simulink model "rev0BB"  (R2017b)
settings: Solver=FixedStepDiscrete  StartTime=0  StopTime=(((preLen+100+dataLenSymbols)*1+pad_first*3)*basePer)  RelTol=1e-3
values from neighbouring files (symbols this model uses):
  ack_stf_len_symbols = length(x_ACK_STF)    [rev0BB_setup.m]
  agc_delay_lag = 32    [rev0BB_setup.m]
  agc_detector_coef = ones(1,agc_detector_taps)./agc_detector_taps    [rev0BB_setup.m]
  agc_on = true    [rev0BB_startup.m]
  agc_sat_low = -agcSaturation    (= -12)    [rev0BB_setup.m]
  agc_sat_up = agcSaturation    (= 12)    [rev0BB_setup.m]
  agcDesired = 0    [rev0BB_setup.m]
  agcExpDomain = agcSaturation    (= 12)    [rev0BB_setup.m]
  agcExpResolution = 2^-5    (= 0.03125)    [rev0BB_setup.m]
  agcPwrAvgNum = 128    [rev0BB_setup.m]
  agcSaturation = 12    [rev0BB_setup.m]
  agcSettleThresh = 0.65    [rev0BB_setup.m]
  agcStep = 2^-8    (= 0.00390625)    [rev0BB_setup.m]
  atanDomain = 5    [rev0BB_setup.m]
  atanDomainTiming = 256    [rev0BB_setup.m]
  atanResolution = 2^-9    (= 0.001953125)    [rev0BB_setup.m]
  atanResolutionTiming = 2^-5    (= 0.03125)    [rev0BB_setup.m]
  averaging_num = ones(1, averaging_samples)    [rev0BB_setup.m]
  averaging_samples = 128    [rev0BB_setup.m]
  awgnSeed = abs(dBSnrRange(dBSnrInd)*1000+trial+10000000)    [plotBer.m]    (also in rev0BB_startup.m = 67)
  basePer = 1/baseFreq    (= 5e-08)    [rev0BB_setup.m]
  bitsPerSymbolHeader = log2(radixHeader)    [rev0BB_setup.m]
  bitsPerSymbolMax = log2(radixMax)    [rev0BB_setup.m]
  cal_sig_i_mult = 1.0    (= 1)    [rev0BB_startup.m]
  cal_sig_i_offset = 0.0    (= 0)    [rev0BB_startup.m]
  cal_sig_q_mult = 1.0    (= 1)    [rev0BB_startup.m]
  cal_sig_q_offset = 0.0    (= 0)    [rev0BB_startup.m]
  cefEarlyWarning = 256    [rev0BB_setup.m]
  cefLen = length(x_CEF)    [rev0BB_setup.m]
  channelFIR = zeros(1, round(maxSampleDelay)+1)    [rev0BB_startup.m]
  coarseCFOAdaptDelay = 1    [rev0BB_setup.m]
  cr_i = 0.020    (= 0.02)    [rev0BB_setup.m]
  cr_i_preamp = 2^-9    (= 0.001953125)    [rev0BB_setup.m]
  cr_int1_sat_low = -cr_integrator1_saturation    (= -0.6)    [rev0BB_setup.m]
  cr_int1_sat_up = cr_integrator1_saturation    (= 0.6)    [rev0BB_setup.m]
  cr_integrator1_decay = 1    [rev0BB_setup.m]
  cr_integrator1_saturation = 0.6    [rev0BB_setup.m]
  cr_mult_pipeline = 0    [rev0BB_setup.m]
  cr_p = 0.015    [rev0BB_setup.m]
  cr_sat2_low = -cr_saturation2    (= -0.6)    [rev0BB_setup.m]
  cr_sat2_up = cr_saturation2    (= 0.6)    [rev0BB_setup.m]
  cr_smooth_num = (1/cr_smooth_samples).*ones(1, cr_smooth_samples)    [rev0BB_setup.m]
  D_128 = [ 1,  8,  2,  4, 16, 32, 64]    [golay.m]    (also in rev0BB_setup.m)
  D_32 = [ 1,  4,  8,  2, 16]    [golay.m]    (also in rev0BB_setup.m)
  dataLenSymbols = header_len_bytes*8/bitsPerSymbolHeader + frame_len_bytes*8/bitsPerSymbol    [rev0BB_setup.m]
  default_channel = 3    [rev0BB_setup.m]
  dmm_coefs = ones(1,dmm_samples)./dmm_samples    [rev0BB_setup.m]
  dst_field_len = 8    [rev0BB_setup.m]
  expDomain = 3.3    [rev0BB_setup.m]
  expResolution = 2^-5    (= 0.03125)    [rev0BB_setup.m]
  expTol = .1    (= 0.1)    [rev0BB_setup.m]
  flush_delay = regular_pipeline*2+mult_pipeline+4    (= 4)    [rev0BB_setup.m]
  frac_lut_domain = 256    [rev0BB_setup.m]
  frac_lut_domain_cr = 64    [rev0BB_setup.m]
  frac_lut_range_max = 512    [rev0BB_setup.m]
  frac_lut_range_max_coarse_cfo = 127    [rev0BB_setup.m]
  frac_lut_range_max_cr = 127    [rev0BB_setup.m]
  frac_lut_range_min = -frac_lut_range_max    (= -512)    [rev0BB_setup.m]
  frac_lut_range_min_coarse_cfo = -frac_lut_range_max_coarse_cfo    (= -127)    [rev0BB_setup.m]
  frac_lut_range_min_cr = -frac_lut_range_max_cr    (= -127)    [rev0BB_setup.m]
  frac_lut_table_breaks = -frac_lut_domain:frac_lut_res:(frac_lut_domain-1)    [rev0BB_setup.m]
  frac_lut_table_breaks_coarse_cfo = -frac_lut_domain_coarse_cfo:frac_lut_res_coarse_cfo:(frac_lut_domain_coarse_cfo-1)    [rev0BB_setup.m]
  frac_lut_table_breaks_cr = -frac_lut_domain_cr:frac_lut_res_cr:(frac_lut_domain_cr-1)    [rev0BB_setup.m]
  frac_lut_table_data = 1./frac_lut_table_breaks    [rev0BB_setup.m]
  frac_lut_table_data_coarse_cfo = 1./frac_lut_table_breaks_coarse_cfo    [rev0BB_setup.m]
  frac_lut_table_data_cr = 1./frac_lut_table_breaks_cr    [rev0BB_setup.m]
  freeze_en_agc = true    [rev0BB_startup.m]
  freeze_en_cr_int1 = false    [rev0BB_startup.m]
  freeze_en_cr_int2 = false    [rev0BB_startup.m]
  freeze_en_cr_phase = false    [rev0BB_startup.m]
  freeze_en_tr_int1 = false    [rev0BB_startup.m]
  freeze_en_tr_int2 = false    [rev0BB_startup.m]
  freeze_en_tr_phase = false    [rev0BB_startup.m]
  freeze_on_cef_done = true    [rev0BB_startup.m]
  freeze_on_stf_done = false    [rev0BB_startup.m]
  freeze_on_valid = true    [rev0BB_startup.m]
  golay_type = 32    [rev0BB_setup.m]
  guardInt = int16(4)    [rev0BB_setup.m]
  guardTol = int16(5)    [rev0BB_setup.m]
  header_len_bytes = 8    [rev0BB_setup.m]
  lineWidth = 60    [rev0BB_setup.m]
  lmsEqDepth = 38    [rev0BB_setup.m]
  lmsStep_init = 0.006    [rev0BB_setup.m]
  lmsStep_meta = (lmsStep_final - lmsStep_init)/cefLen    [rev0BB_setup.m]
  lnDomain = 16    [rev0BB_setup.m]
  lnResolution = 2^-5    (= 0.03125)    [rev0BB_setup.m]
  local_node_id = 2    [rev0BB_startup.m]
  maxMsgSize = length(xSpectrum_PRE)+dataLenSymbols+300    [rev0BB_setup.m]
  minSTFPeaks = 3    [rev0BB_setup.m]
  mod_scheme_len_bytes = 1    [rev0BB_setup.m]
  modBPS = [1, 2, 4]    [rev0BB_setup.m]
  modKeys = [0, 1, 2]    [rev0BB_setup.m]
  mult_pipeline = 0    [rev0BB_setup.m]
  overSampleFreq = 80e6    (= 80000000)    [rev0BB_setup.m]
  overSamplePer = 1/overSampleFreq    (= 1.25e-08)    [rev0BB_setup.m]
  pad_first = 1000    [createTestVectors.m]
  post_cr_i_offset = 0    [rev0BB_startup.m]
  post_cr_q_offset = 0    [rev0BB_startup.m]
  preambleSequentialDetect = 2    [rev0BB_setup.m]
  preLen = length(x_PRE)    [rev0BB_setup.m]
  qam16_demod_scale_factor = qam16_hdl_distance/qam16_power_normalized_distance    [rev0BB_setup.m]
  rcRxFilt = [0.000303163120401141 -0.00118915940834234 -0.00187387637177 -0.00124167532697737 0.00029186889076529 0.00164526160586517 0.00182432050803312 0.000652133621739543 -0.00105668254004908 -0.00204011570659167 -0.00150058088768918 0.00026138356356816 0.0019831869994874 0.00231075800085521 0.000821993419120097 -0.00154687337975486 -0.00305430783933469 -0.00238186490079127 0.000301216962040692 0.00325307 ...(+2001 chars)    [rev0BB_setup.m]
  rcTxFilt = [0.000303163120401141 -0.00118915940834234 -0.00187387637177 -0.00124167532697737 0.00029186889076529 0.00164526160586517 0.00182432050803312 0.000652133621739543 -0.00105668254004908 -0.00204011570659167 -0.00150058088768918 0.00026138356356816 0.0019831869994874 0.00231075800085521 0.000821993419120097 -0.00154687337975486 -0.00305430783933469 -0.00238186490079127 0.000301216962040692 0.00325307 ...(+2001 chars)    [rev0BB_setup.m]
  regular_pipeline = 0    [rev0BB_setup.m]
  rx_gain = 1    [rev0BB_setup.m]
  rx_gain_i = 1    [rev0BB_setup.m]
  rx_gain_q = 1    [rev0BB_setup.m]
  rx_impare_i_offset = 0    [rev0BB_startup.m]
  rx_impare_i_scale = 1    [rev0BB_startup.m]
  rx_impare_q_offset = 0    [rev0BB_startup.m]
  rx_impare_q_scale = 1    [rev0BB_startup.m]
  rx_offset_correction_i = 0    [rev0BB_startup.m]
  rx_offset_correction_q = 0    [rev0BB_startup.m]
  sin_source_amp = 1    [rev0BB_setup.m]
  sin_source_freq = 250e6/16    (= 15625000)    [rev0BB_setup.m]
  slowPer = overSamplePer*slowSample    (= 2.5e-08)    [rev0BB_setup.m]
  std_pkt_type = 0    [rev0BB_setup.m]
  stfLen = length(x_STF)    [rev0BB_setup.m]
  testMsg = cat(1, xCTRL_PRE_adj, header, payload)    [plotBer.m]
  timing_i = 0.25    [rev0BB_setup.m]
  ... (+25 more)
undefined symbols (not defined in the file or in its folder): cr_integrator2_saturation, doppler, i, magnitude, useFadingChannel
libraries: helperLib x128, simulink x90, golayLib x34, dspsigops x32, commfilt2 x27, commdigbbndpm3 x8, hdlsllib x6, dsparch4 x4, commdigbbndam3 x4, commchan3 x2, commrflib2 x2, commcrc2 x2
(part 4 of 10)

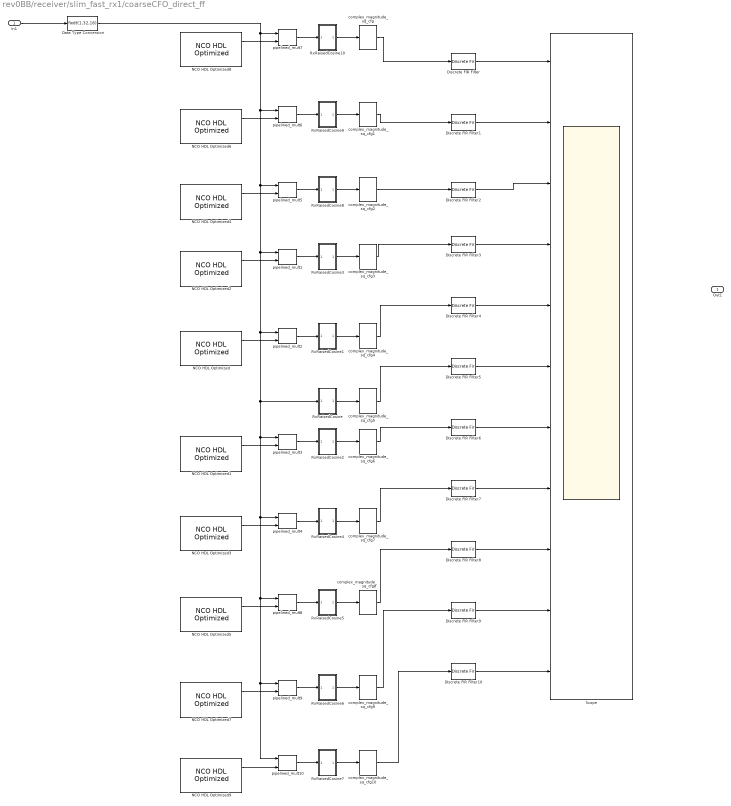
== system rev0BB/receiver/slim_fast_rx1/coarseCFO_direct_ff ==
  In1 : Inport
  Data Type Conversion : DataTypeConversion  OutDataTypeStr=fixdt(1,32,16)
  Discrete FIR Filter{,1..10} (11 alike) : DiscreteFir  Coefficients=ones(1,512)./512
  NCO HDL Optimized : dspsigops/NCO HDL Optimized  PhaseIncrementSource=Property  PhaseIncrement=floor(1000*2^17/overSampleFreq)  PhaseOffsetSource=Property  PhaseOffset=0  DitherSource=Property  NumDitherBits=4  PhaseQuantization=on  NumQuantizerAccumulatorBits=17  LUTCompress=on  ResetAction=off  ValidInputPort=off  Waveform=Complex exponential  PhasePort=off  SimulateUsing=Code generation  AccumulatorWL=21  OutputDataType=Binary point scaling  OutputWL=18  OutputFL=11
      settings: SourceProductName=DSP System Toolbox  SourceProductBaseCode=DS
  NCO HDL Optimized1 : dspsigops/NCO HDL Optimized  PhaseIncrementSource=Property  PhaseIncrement=-floor(1000*2^17/overSampleFreq)  PhaseOffsetSource=Property  PhaseOffset=0  DitherSource=Property  NumDitherBits=4  PhaseQuantization=on  NumQuantizerAccumulatorBits=17  LUTCompress=on  ResetAction=off  ValidInputPort=off  Waveform=Complex exponential  PhasePort=off  SimulateUsing=Code generation  AccumulatorWL=21  OutputDataType=Binary point scaling  OutputWL=18  OutputFL=11
      settings: SourceProductName=DSP System Toolbox  SourceProductBaseCode=DS
  NCO HDL Optimized2 : dspsigops/NCO HDL Optimized  PhaseIncrementSource=Property  PhaseIncrement=floor(2000*2^17/overSampleFreq)  PhaseOffsetSource=Property  PhaseOffset=0  DitherSource=Property  NumDitherBits=4  PhaseQuantization=on  NumQuantizerAccumulatorBits=17  LUTCompress=on  ResetAction=off  ValidInputPort=off  Waveform=Complex exponential  PhasePort=off  SimulateUsing=Code generation  AccumulatorWL=21  OutputDataType=Binary point scaling  OutputWL=18  OutputFL=11
      settings: SourceProductName=DSP System Toolbox  SourceProductBaseCode=DS
  NCO HDL Optimized3 : dspsigops/NCO HDL Optimized  PhaseIncrementSource=Property  PhaseIncrement=-floor(2000*2^17/overSampleFreq)  PhaseOffsetSource=Property  PhaseOffset=0  DitherSource=Property  NumDitherBits=4  PhaseQuantization=on  NumQuantizerAccumulatorBits=17  LUTCompress=on  ResetAction=off  ValidInputPort=off  Waveform=Complex exponential  PhasePort=off  SimulateUsing=Code generation  AccumulatorWL=21  OutputDataType=Binary point scaling  OutputWL=18  OutputFL=11
      settings: SourceProductName=DSP System Toolbox  SourceProductBaseCode=DS
  NCO HDL Optimized4 : dspsigops/NCO HDL Optimized  PhaseIncrementSource=Property  PhaseIncrement=floor(3000*2^17/overSampleFreq)  PhaseOffsetSource=Property  PhaseOffset=0  DitherSource=Property  NumDitherBits=4  PhaseQuantization=on  NumQuantizerAccumulatorBits=17  LUTCompress=on  ResetAction=off  ValidInputPort=off  Waveform=Complex exponential  PhasePort=off  SimulateUsing=Code generation  AccumulatorWL=21  OutputDataType=Binary point scaling  OutputWL=18  OutputFL=11
      settings: SourceProductName=DSP System Toolbox  SourceProductBaseCode=DS
  NCO HDL Optimized5 : dspsigops/NCO HDL Optimized  PhaseIncrementSource=Property  PhaseIncrement=floor(-3000*2^17/overSampleFreq)  PhaseOffsetSource=Property  PhaseOffset=0  DitherSource=Property  NumDitherBits=4  PhaseQuantization=on  NumQuantizerAccumulatorBits=17  LUTCompress=on  ResetAction=off  ValidInputPort=off  Waveform=Complex exponential  PhasePort=off  SimulateUsing=Code generation  AccumulatorWL=21  OutputDataType=Binary point scaling  OutputWL=18  OutputFL=11
      settings: SourceProductName=DSP System Toolbox  SourceProductBaseCode=DS
  NCO HDL Optimized6 : dspsigops/NCO HDL Optimized  PhaseIncrementSource=Property  PhaseIncrement=floor(4000*2^17/overSampleFreq)  PhaseOffsetSource=Property  PhaseOffset=0  DitherSource=Property  NumDitherBits=4  PhaseQuantization=on  NumQuantizerAccumulatorBits=17  LUTCompress=on  ResetAction=off  ValidInputPort=off  Waveform=Complex exponential  PhasePort=off  SimulateUsing=Code generation  AccumulatorWL=21  OutputDataType=Binary point scaling  OutputWL=18  OutputFL=11
      settings: SourceProductName=DSP System Toolbox  SourceProductBaseCode=DS
  NCO HDL Optimized7 : dspsigops/NCO HDL Optimized  PhaseIncrementSource=Property  PhaseIncrement=-floor(4000*2^17/overSampleFreq)  PhaseOffsetSource=Property  PhaseOffset=0  DitherSource=Property  NumDitherBits=4  PhaseQuantization=on  NumQuantizerAccumulatorBits=17  LUTCompress=on  ResetAction=off  ValidInputPort=off  Waveform=Complex exponential  PhasePort=off  SimulateUsing=Code generation  AccumulatorWL=21  OutputDataType=Binary point scaling  OutputWL=18  OutputFL=11
      settings: SourceProductName=DSP System Toolbox  SourceProductBaseCode=DS
  NCO HDL Optimized8 : dspsigops/NCO HDL Optimized  PhaseIncrementSource=Property  PhaseIncrement=floor(5000*2^17/overSampleFreq)  PhaseOffsetSource=Property  PhaseOffset=0  DitherSource=Property  NumDitherBits=4  PhaseQuantization=on  NumQuantizerAccumulatorBits=17  LUTCompress=on  ResetAction=off  ValidInputPort=off  Waveform=Complex exponential  PhasePort=off  SimulateUsing=Code generation  AccumulatorWL=21  OutputDataType=Binary point scaling  OutputWL=18  OutputFL=11
      settings: SourceProductName=DSP System Toolbox  SourceProductBaseCode=DS
  NCO HDL Optimized9 : dspsigops/NCO HDL Optimized  PhaseIncrementSource=Property  PhaseIncrement=-floor(5000*2^17/overSampleFreq)  PhaseOffsetSource=Property  PhaseOffset=0  DitherSource=Property  NumDitherBits=4  PhaseQuantization=on  NumQuantizerAccumulatorBits=17  LUTCompress=on  ResetAction=off  ValidInputPort=off  Waveform=Complex exponential  PhasePort=off  SimulateUsing=Code generation  AccumulatorWL=21  OutputDataType=Binary point scaling  OutputWL=18  OutputFL=11
      settings: SourceProductName=DSP System Toolbox  SourceProductBaseCode=DS
  RxRaisedCosine : Subsystem
  RxRaisedCosine1 : Subsystem
  RxRaisedCosine10 : Subsystem
  RxRaisedCosine2 : Subsystem
  RxRaisedCosine3 : Subsystem
  RxRaisedCosine4 : Subsystem
  RxRaisedCosine5 : Subsystem
  RxRaisedCosine6 : Subsystem
  RxRaisedCosine7 : Subsystem
  RxRaisedCosine8 : Subsystem
  RxRaisedCosine9 : Subsystem
  Scope : Scope  NumInputPorts=11
  complex_magnitude_sq_cfg{,1..10} (11 alike) : helperLib/complex_magnitude_sq_cfg  mult=mult_pipeline  pipe=regular_pipeline
  pipelined_mult{1..10} (10 alike) : helperLib/pipelined_mult  d=wide_mult_pipeline
  Out1 : Outport
  wires:
  NCO HDL Optimized/1 -> pipelined_mult2/2
  NCO HDL Optimized1/1 -> pipelined_mult3/2
  pipelined_mult3/1 -> RxRaisedCosine2/1(In2)
  pipelined_mult2/1 -> RxRaisedCosine1/1(In2)
  NCO HDL Optimized6/1 -> pipelined_mult6/2
  NCO HDL Optimized4/1 -> pipelined_mult5/2
  NCO HDL Optimized2/1 -> pipelined_mult1/2
  pipelined_mult1/1 -> RxRaisedCosine3/1(In2)
  NCO HDL Optimized8/1 -> pipelined_mult7/2
  In1/1 -> Data Type Conversion/1
  NCO HDL Optimized3/1 -> pipelined_mult4/2
  NCO HDL Optimized5/1 -> pipelined_mult8/2
  NCO HDL Optimized7/1 -> pipelined_mult9/2
  NCO HDL Optimized9/1 -> pipelined_mult10/2
  pipelined_mult4/1 -> RxRaisedCosine4/1(In2)
  pipelined_mult8/1 -> RxRaisedCosine5/1(In2)
  pipelined_mult9/1 -> RxRaisedCosine6/1(In2)
  pipelined_mult10/1 -> RxRaisedCosine7/1(In2)
  pipelined_mult5/1 -> RxRaisedCosine8/1(In2)
  pipelined_mult6/1 -> RxRaisedCosine9/1(In2)
  pipelined_mult7/1 -> RxRaisedCosine10/1(In2)
  RxRaisedCosine10/1(Out2) -> complex_magnitude_sq_cfg/1
  RxRaisedCosine9/1(Out2) -> complex_magnitude_sq_cfg1/1
  RxRaisedCosine8/1(Out2) -> complex_magnitude_sq_cfg2/1
  RxRaisedCosine3/1(Out2) -> complex_magnitude_sq_cfg3/1
  RxRaisedCosine1/1(Out2) -> complex_magnitude_sq_cfg4/1
  RxRaisedCosine/1(Out2) -> complex_magnitude_sq_cfg5/1
  RxRaisedCosine2/1(Out2) -> complex_magnitude_sq_cfg6/1
  RxRaisedCosine4/1(Out2) -> complex_magnitude_sq_cfg7/1
  RxRaisedCosine5/1(Out2) -> complex_magnitude_sq_cfg8/1
  RxRaisedCosine6/1(Out2) -> complex_magnitude_sq_cfg9/1
  RxRaisedCosine7/1(Out2) -> complex_magnitude_sq_cfg10/1
  complex_magnitude_sq_cfg/1 -> Discrete FIR Filter/1
  complex_magnitude_sq_cfg1/1 -> Discrete FIR Filter1/1
  complex_magnitude_sq_cfg2/1 -> Discrete FIR Filter2/1
  complex_magnitude_sq_cfg3/1 -> Discrete FIR Filter3/1
  complex_magnitude_sq_cfg4/1 -> Discrete FIR Filter4/1
  complex_magnitude_sq_cfg5/1 -> Discrete FIR Filter5/1
  complex_magnitude_sq_cfg6/1 -> Discrete FIR Filter6/1
  complex_magnitude_sq_cfg7/1 -> Discrete FIR Filter7/1
  complex_magnitude_sq_cfg8/1 -> Discrete FIR Filter8/1
  complex_magnitude_sq_cfg9/1 -> Discrete FIR Filter9/1
  complex_magnitude_sq_cfg10/1 -> Discrete FIR Filter10/1
  Data Type Conversion/1 -> pipelined_mult7/1, pipelined_mult6/1, pipelined_mult5/1, pipelined_mult1/1, RxRaisedCosine/1(In2), pipelined_mult10/1, pipelined_mult9/1, pipelined_mult8/1, pipelined_mult4/1, pipelined_mult3/1, pipelined_mult2/1
  Discrete FIR Filter/1 -> Scope/1
  Discrete FIR Filter1/1 -> Scope/2
  Discrete FIR Filter2/1 -> Scope/3
  Discrete FIR Filter3/1 -> Scope/4
  Discrete FIR Filter4/1 -> Scope/5
  Discrete FIR Filter5/1 -> Scope/6
  Discrete FIR Filter6/1 -> Scope/7
  Discrete FIR Filter7/1 -> Scope/8
  Discrete FIR Filter8/1 -> Scope/9
  Discrete FIR Filter9/1 -> Scope/10
  Discrete FIR Filter10/1 -> Scope/11

== system rev0BB/receiver/slim_fast_rx1/coarseCFO_ff ==
  note: The frequency estemator is derived in Ch 8.2.2 (Pg 457-462) in
      | Digital Communication Recievers: Syncronization, Channel Estimation, and Signal Processing by Meyr et al.
  SignalIn : Inport
  Coarse_CFO_EST : Scope
  Complex to Real-Imag : ComplexToRealImag
  Constant : Constant  Value=0  OutDataTypeStr=int16
  Constant1 : Constant  Value=true  OutDataTypeStr=boolean
  Data Type Conversion : DataTypeConversion  OutDataTypeStr=double
  Data Type Conversion1 : DataTypeConversion  OutDataTypeStr=double
  Delay : Delay  DelayLength=1  InitialCondition=0
  Discrete FIR Filter : DiscreteFir  Coefficients=ones(1, 4096)  AccumDataTypeStr=Inherit: Same as product output
  Gain : Gain  Gain=overSampleFreq/(2*pi)
  NCO HDL Optimized : dspsigops/NCO HDL Optimized  PhaseIncrementSource=Input port  PhaseIncrement=100  PhaseOffsetSource=Property  PhaseOffset=0  DitherSource=Property  NumDitherBits=4  PhaseQuantization=on  NumQuantizerAccumulatorBits=12  LUTCompress=on  ResetAction=off  ValidInputPort=on  Waveform=Complex exponential  PhasePort=off  SimulateUsing=Code generation  AccumulatorWL=14  OutputDataType=Binary point scaling  OutputWL=14  OutputFL=11
      settings: SourceProductName=DSP System Toolbox  SourceProductBaseCode=DS
  Product : Product
  Trigonometric Function : Trigonometry  Operator=atan2
  complex_conj : helperLib/complex_conj
  pipeline_delay : Delay  DelayLength=regular_pipeline
  pipelined_mult1 : helperLib/pipelined_mult  d=wide_mult_pipeline
  SignalOut : Outport
  wires:
  NCO HDL Optimized/1 -> pipelined_mult1/2
  SignalIn/1 -> pipeline_delay/1, pipelined_mult1/1
  pipelined_mult1/1 -> SignalOut/1
  Constant1/1 -> NCO HDL Optimized/2
  Delay/1 -> complex_conj/1
  pipeline_delay/1 -> Data Type Conversion/1, Delay/1
  Constant/1 -> NCO HDL Optimized/1
  Trigonometric Function/1 -> Gain/1
  complex_conj/1 -> Data Type Conversion1/1
  Data Type Conversion1/1 -> Product/1
  Data Type Conversion/1 -> Product/2
  Product/1 -> Discrete FIR Filter/1
  Discrete FIR Filter/1 -> Complex to Real-Imag/1
  Complex to Real-Imag/2 -> Trigonometric Function/1
  Complex to Real-Imag/1 -> Trigonometric Function/2
  Gain/1 -> Coarse_CFO_EST/1

== system rev0BB/receiver/slim_fast_rx2/AGC ==
  note: Intentionally let width grow due to distinct chance of overflow
  In : Inport
  Desired : Inport  Port=2
  Step : Inport  Port=3
  freeze : Inport  Port=4  OutDataTypeStr=boolean
  agc_sat_up : Inport  Port=5
  agc_sat_low : Inport  Port=6
  Bit Shift : hdlsllib/Logic and Bit Operations/Bit Shift  Commented=on  mode=Shift Left Logical  N=1
      settings: SourceProductName=HDL Coder  SourceProductBaseCode=HD
  Constant : Constant  Value=0  OutDataTypeStr=Inherit: Inherit via back propagation  SampleTime=-1
  Data Type Duplicate : DataTypeDuplicate  Commented=on
  Data Type Duplicate1 : DataTypeDuplicate
  Data Type Conversion1 : DataTypeConversion  OutDataTypeStr=fixdt(1,38,18)
  Delay : Delay  DelayLength=1  InitialCondition=0
  Delay1 : Delay  DelayLength=1  InitialCondition=0
  Discrete FIR Filter : DiscreteFir  FilterStructure=Direct form transposed  Coefficients=agc_detector_coef  InputProcessing=Columns as channels (frame based)  OutDataTypeStr=Inherit: Same as input
  Product : Product  Commented=on
  Saturation : Saturate  Commented=on  UpperLimit=agcSaturation  LowerLimit=-agcSaturation
  Saturation Dynamic : simulink/Discontinuities/Saturation Dynamic  OutMin=[]  OutMax=[]  OutDataTypeStr=Inherit: Same as second input  OutDataType=fixdt(1, 16)  OutScaling=2^-10  DoSatur=off
  Sum : Sum  Inputs=-+
  Sum1 : Sum  Inputs=|++
  Switch : Switch  Criteria=u2 > Threshold
  Switch1 : Switch  Criteria=u2 > Threshold
  complex_magnitude_sq_cfg : helperLib/complex_magnitude_sq_cfg  mult=wide_mult_pipeline  pipe=regular_pipeline
  exp : Subsystem
  exp1 : Subsystem  Commented=on
  ln1 : Subsystem
  mult_delay1 : Delay  Commented=on  DelayLength=wide_mult_pipeline
  pipeline_delay{,1..2,4,7..13} (11 alike) : Delay  DelayLength=regular_pipeline
  pipeline_delay3 : Delay  Commented=on  DelayLength=regular_pipeline
  pipeline_delay5 : Delay  Commented=on  DelayLength=regular_pipeline
  pipeline_delay6 : Delay  DelayLength=regular_pipeline*2
  pipelined_mult2 : helperLib/pipelined_mult  d=wide_mult_pipeline
  Correction : Outport
  LnPwr : Outport  Port=2
  wires:
  In/1 -> Data Type Conversion1/1
  Data Type Conversion1/1 -> pipeline_delay6/1
  complex_magnitude_sq_cfg/1 -> pipeline_delay9/1
  ln1/1(Out) -> pipeline_delay10/1
  Sum/1 -> pipeline_delay/1
  pipeline_delay/1 -> pipelined_mult2/2
  pipeline_delay7/1 -> pipelined_mult2/1
  Bit Shift/1 -> pipeline_delay3/1
  Sum1/1 -> Delay/1
  exp1/1(Out) -> pipeline_delay5/1
  pipeline_delay5/1 -> Data Type Duplicate/2, Product/2
  exp/1(Out) -> pipeline_delay4/1
  pipeline_delay4/1 -> Data Type Duplicate1/1, Correction/1
  Step/1 -> pipeline_delay7/1
  Desired/1 -> pipeline_delay8/1
  pipeline_delay10/1 -> LnPwr/1, Sum/1
  pipeline_delay2/1 -> exp/1(In)
  pipeline_delay3/1 -> exp1/1(In)
  pipeline_delay8/1 -> Sum/2
  pipeline_delay1/1 -> Data Type Duplicate1/2, ln1/2(data_type), Data Type Duplicate/1, Product/1, ln1/1(In)
  Saturation Dynamic/1 -> Sum1/2, Switch/3
  pipelined_mult2/1 -> Switch1/3
  Product/1 -> mult_delay1/1
  Switch/1 -> Bit Shift/1, pipeline_delay2/1, Delay1/1
  freeze/1 -> pipeline_delay13/1
  Delay1/1 -> Switch/1
  agc_sat_up/1 -> pipeline_delay11/1
  agc_sat_low/1 -> pipeline_delay12/1
  Delay/1 -> Saturation Dynamic/2
  pipeline_delay9/1 -> Discrete FIR Filter/1
  Discrete FIR Filter/1 -> pipeline_delay1/1
  pipeline_delay6/1 -> complex_magnitude_sq_cfg/1
  pipeline_delay11/1 -> Saturation Dynamic/1
  pipeline_delay12/1 -> Saturation Dynamic/3
  pipeline_delay13/1 -> Switch1/2, Switch/2
  Switch1/1 -> Sum1/1
  Constant/1 -> Switch1/1

== system rev0BB/receiver/slim_fast_rx2/Golay Correlator 128 ==
  In : Inport
  GolayCoralatorBase_fp : golayLib/GolayCoralatorBase_fp  dSub=D_128(1)*4  wSub=W_128(1)  mult=0
  GolayCoralatorBase_fp1 : golayLib/GolayCoralatorBase_fp  dSub=D_128(2)*4  wSub=W_128(2)  mult=0
  GolayCoralatorBase_fp2 : golayLib/GolayCoralatorBase_fp  dSub=D_128(3)*4  wSub=W_128(3)  mult=0
  GolayCoralatorBase_fp3 : golayLib/GolayCoralatorBase_fp  dSub=D_128(4)*4  wSub=W_128(4)  mult=0
  GolayCoralatorBase_fp4 : golayLib/GolayCoralatorBase_fp  dSub=D_128(5)*4  wSub=W_128(5)  mult=0
  GolayCoralatorBase_fp5 : golayLib/GolayCoralatorBase_fp  dSub=D_128(6)*4  wSub=W_128(6)  mult=0
  GolayCoralatorBase_fp6 : golayLib/GolayCoralatorBase_fp  dSub=D_128(7)*4  wSub=W_128(7)  mult=0
  pipeline_delay{,1..13} (14 alike) : Delay  DelayLength=regular_pipeline
  Ca : Outport
  Cb : Outport  Port=2
  wires:
  GolayCoralatorBase_fp/1 -> pipeline_delay/1
  GolayCoralatorBase_fp/2 -> pipeline_delay1/1
  GolayCoralatorBase_fp1/1 -> pipeline_delay2/1
  GolayCoralatorBase_fp1/2 -> pipeline_delay3/1
  GolayCoralatorBase_fp4/1 -> pipeline_delay8/1
  GolayCoralatorBase_fp2/1 -> pipeline_delay4/1
  GolayCoralatorBase_fp2/2 -> pipeline_delay5/1
  GolayCoralatorBase_fp3/1 -> pipeline_delay6/1
  GolayCoralatorBase_fp3/2 -> pipeline_delay7/1
  GolayCoralatorBase_fp5/2 -> pipeline_delay11/1
  GolayCoralatorBase_fp5/1 -> pipeline_delay10/1
  GolayCoralatorBase_fp6/1 -> pipeline_delay12/1
  In/1 -> GolayCoralatorBase_fp/2, GolayCoralatorBase_fp/1
  pipeline_delay/1 -> GolayCoralatorBase_fp1/1
  pipeline_delay1/1 -> GolayCoralatorBase_fp1/2
  pipeline_delay2/1 -> GolayCoralatorBase_fp2/1
  pipeline_delay3/1 -> GolayCoralatorBase_fp2/2
  pipeline_delay4/1 -> GolayCoralatorBase_fp3/1
  pipeline_delay6/1 -> GolayCoralatorBase_fp4/1
  pipeline_delay8/1 -> GolayCoralatorBase_fp5/1
  pipeline_delay10/1 -> GolayCoralatorBase_fp6/1
  pipeline_delay12/1 -> Ca/1
  pipeline_delay13/1 -> Cb/1
  pipeline_delay5/1 -> GolayCoralatorBase_fp3/2
  pipeline_delay7/1 -> GolayCoralatorBase_fp4/2
  GolayCoralatorBase_fp4/2 -> pipeline_delay9/1
  pipeline_delay9/1 -> GolayCoralatorBase_fp5/2
  pipeline_delay11/1 -> GolayCoralatorBase_fp6/2
  GolayCoralatorBase_fp6/2 -> pipeline_delay13/1

== system rev0BB/receiver/slim_fast_rx2/Golay Correlator 32 ==
  In : Inport
  GolayCoralatorBase_fp : golayLib/GolayCoralatorBase_fp  dSub=D_32(1)*4  wSub=W_32(1)  mult=0
  GolayCoralatorBase_fp1 : golayLib/GolayCoralatorBase_fp  dSub=D_32(2)*4  wSub=W_32(2)  mult=0
  GolayCoralatorBase_fp2 : golayLib/GolayCoralatorBase_fp  dSub=D_32(3)*4  wSub=W_32(3)  mult=0
  GolayCoralatorBase_fp3 : golayLib/GolayCoralatorBase_fp  dSub=D_32(4)*4  wSub=W_32(4)  mult=0
  GolayCoralatorBase_fp4 : golayLib/GolayCoralatorBase_fp  dSub=D_32(5)*4  wSub=W_32(5)  mult=0
  pipeline_delay{,1..13} (14 alike) : Delay  DelayLength=regular_pipeline
  Ca : Outport
  Cb : Outport  Port=2
  wires:
  GolayCoralatorBase_fp/1 -> pipeline_delay/1
  GolayCoralatorBase_fp/2 -> pipeline_delay1/1
  GolayCoralatorBase_fp1/1 -> pipeline_delay2/1
  GolayCoralatorBase_fp1/2 -> pipeline_delay3/1
  GolayCoralatorBase_fp4/1 -> pipeline_delay8/1
  GolayCoralatorBase_fp2/1 -> pipeline_delay4/1
  GolayCoralatorBase_fp2/2 -> pipeline_delay5/1
  GolayCoralatorBase_fp3/1 -> pipeline_delay6/1
  GolayCoralatorBase_fp3/2 -> pipeline_delay7/1
  pipeline_delay9/1 -> pipeline_delay11/1
  pipeline_delay8/1 -> pipeline_delay10/1
  pipeline_delay10/1 -> pipeline_delay12/1
  In/1 -> GolayCoralatorBase_fp/2, GolayCoralatorBase_fp/1
  pipeline_delay/1 -> GolayCoralatorBase_fp1/1
  pipeline_delay1/1 -> GolayCoralatorBase_fp1/2
  pipeline_delay2/1 -> GolayCoralatorBase_fp2/1
  pipeline_delay3/1 -> GolayCoralatorBase_fp2/2
  pipeline_delay4/1 -> GolayCoralatorBase_fp3/1
  pipeline_delay6/1 -> GolayCoralatorBase_fp4/1
  pipeline_delay12/1 -> Ca/1
  pipeline_delay13/1 -> Cb/1
  pipeline_delay5/1 -> GolayCoralatorBase_fp3/2
  pipeline_delay7/1 -> GolayCoralatorBase_fp4/2
  GolayCoralatorBase_fp4/2 -> pipeline_delay9/1
  pipeline_delay11/1 -> pipeline_delay13/1

== system rev0BB/receiver/slim_fast_rx2/RxRaisedCosine1 ==
  In2 : Inport
  Discrete FIR Filter : DiscreteFir  FilterStructure=Direct form transposed  Coefficients=rcRxFilt  AccumDataTypeStr=Inherit: Same as product output
  Raised Cosine Receive Filter : commfilt2/Raised Cosine Receive Filter  Commented=on  filtType=Square root  R=0.2  filtSpan=10  N=4  downFactor=1  downOffset=0  filterGain=1  InputProcessing=Columns as channels (frame based)  RateOptions=Enforce single-rate processing  framing=Mute  checkCoeff=on  variableName=rcRxFilt  currentFiltSpan=10  D=5  inputOffset=0  sampMode=Mute  saveAsFlag=0  rateMode=Downsampling  checkGain=Normalized  launchFVT=on  roundingMode=Floor  overflowMode=off  coeffDataTypeStr=Inherit: Same word length as input  coeffMin=[]  coeffMax=[]  coeffLastDataTypeStr=Inherit: Same word length as input  accumDataTypeStr=Inherit: Same as product output  accumLastDataTypeStr=Inherit: Same as product output  outputDataTypeStr=Inherit: Same as accumulator  outputMin=[]  outputMax=[]  outputLastDataTypeStr=Inherit: Same as accumulator
  Out2 : Outport
  wires:
  Discrete FIR Filter/1 -> Out2/1
  In2/1 -> Discrete FIR Filter/1

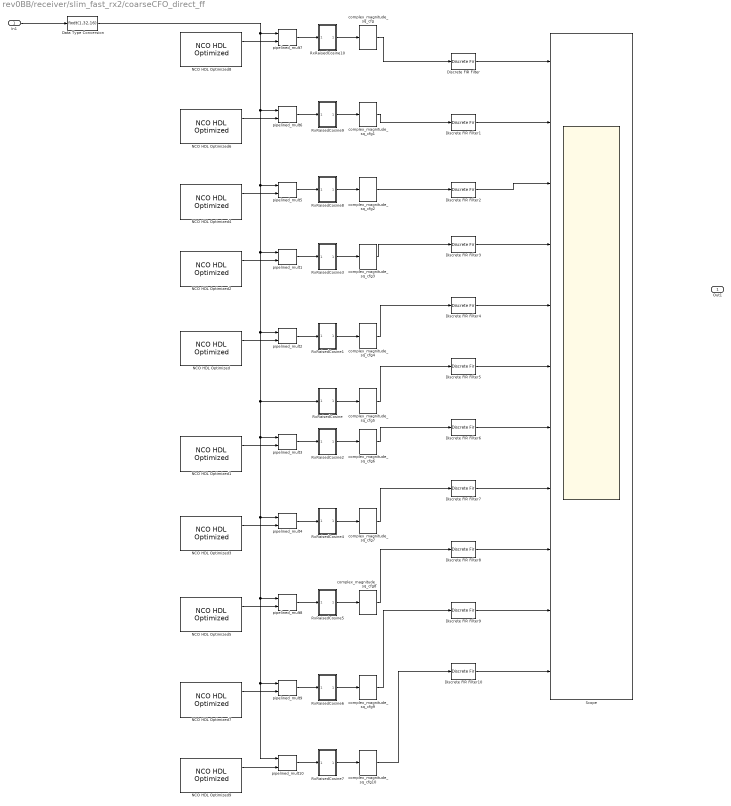
== system rev0BB/receiver/slim_fast_rx2/coarseCFO_direct_ff ==
  In1 : Inport
  Data Type Conversion : DataTypeConversion  OutDataTypeStr=fixdt(1,32,16)
  Discrete FIR Filter{,1..10} (11 alike) : DiscreteFir  Coefficients=ones(1,512)./512
  NCO HDL Optimized : dspsigops/NCO HDL Optimized  PhaseIncrementSource=Property  PhaseIncrement=floor(1000*2^17/overSampleFreq)  PhaseOffsetSource=Property  PhaseOffset=0  DitherSource=Property  NumDitherBits=4  PhaseQuantization=on  NumQuantizerAccumulatorBits=17  LUTCompress=on  ResetAction=off  ValidInputPort=off  Waveform=Complex exponential  PhasePort=off  SimulateUsing=Code generation  AccumulatorWL=21  OutputDataType=Binary point scaling  OutputWL=18  OutputFL=11
      settings: SourceProductName=DSP System Toolbox  SourceProductBaseCode=DS
  NCO HDL Optimized1 : dspsigops/NCO HDL Optimized  PhaseIncrementSource=Property  PhaseIncrement=-floor(1000*2^17/overSampleFreq)  PhaseOffsetSource=Property  PhaseOffset=0  DitherSource=Property  NumDitherBits=4  PhaseQuantization=on  NumQuantizerAccumulatorBits=17  LUTCompress=on  ResetAction=off  ValidInputPort=off  Waveform=Complex exponential  PhasePort=off  SimulateUsing=Code generation  AccumulatorWL=21  OutputDataType=Binary point scaling  OutputWL=18  OutputFL=11
      settings: SourceProductName=DSP System Toolbox  SourceProductBaseCode=DS
  NCO HDL Optimized2 : dspsigops/NCO HDL Optimized  PhaseIncrementSource=Property  PhaseIncrement=floor(2000*2^17/overSampleFreq)  PhaseOffsetSource=Property  PhaseOffset=0  DitherSource=Property  NumDitherBits=4  PhaseQuantization=on  NumQuantizerAccumulatorBits=17  LUTCompress=on  ResetAction=off  ValidInputPort=off  Waveform=Complex exponential  PhasePort=off  SimulateUsing=Code generation  AccumulatorWL=21  OutputDataType=Binary point scaling  OutputWL=18  OutputFL=11
      settings: SourceProductName=DSP System Toolbox  SourceProductBaseCode=DS
  NCO HDL Optimized3 : dspsigops/NCO HDL Optimized  PhaseIncrementSource=Property  PhaseIncrement=-floor(2000*2^17/overSampleFreq)  PhaseOffsetSource=Property  PhaseOffset=0  DitherSource=Property  NumDitherBits=4  PhaseQuantization=on  NumQuantizerAccumulatorBits=17  LUTCompress=on  ResetAction=off  ValidInputPort=off  Waveform=Complex exponential  PhasePort=off  SimulateUsing=Code generation  AccumulatorWL=21  OutputDataType=Binary point scaling  OutputWL=18  OutputFL=11
      settings: SourceProductName=DSP System Toolbox  SourceProductBaseCode=DS
  NCO HDL Optimized4 : dspsigops/NCO HDL Optimized  PhaseIncrementSource=Property  PhaseIncrement=floor(3000*2^17/overSampleFreq)  PhaseOffsetSource=Property  PhaseOffset=0  DitherSource=Property  NumDitherBits=4  PhaseQuantization=on  NumQuantizerAccumulatorBits=17  LUTCompress=on  ResetAction=off  ValidInputPort=off  Waveform=Complex exponential  PhasePort=off  SimulateUsing=Code generation  AccumulatorWL=21  OutputDataType=Binary point scaling  OutputWL=18  OutputFL=11
      settings: SourceProductName=DSP System Toolbox  SourceProductBaseCode=DS
  NCO HDL Optimized5 : dspsigops/NCO HDL Optimized  PhaseIncrementSource=Property  PhaseIncrement=floor(-3000*2^17/overSampleFreq)  PhaseOffsetSource=Property  PhaseOffset=0  DitherSource=Property  NumDitherBits=4  PhaseQuantization=on  NumQuantizerAccumulatorBits=17  LUTCompress=on  ResetAction=off  ValidInputPort=off  Waveform=Complex exponential  PhasePort=off  SimulateUsing=Code generation  AccumulatorWL=21  OutputDataType=Binary point scaling  OutputWL=18  OutputFL=11
      settings: SourceProductName=DSP System Toolbox  SourceProductBaseCode=DS
  NCO HDL Optimized6 : dspsigops/NCO HDL Optimized  PhaseIncrementSource=Property  PhaseIncrement=floor(4000*2^17/overSampleFreq)  PhaseOffsetSource=Property  PhaseOffset=0  DitherSource=Property  NumDitherBits=4  PhaseQuantization=on  NumQuantizerAccumulatorBits=17  LUTCompress=on  ResetAction=off  ValidInputPort=off  Waveform=Complex exponential  PhasePort=off  SimulateUsing=Code generation  AccumulatorWL=21  OutputDataType=Binary point scaling  OutputWL=18  OutputFL=11
      settings: SourceProductName=DSP System Toolbox  SourceProductBaseCode=DS
  NCO HDL Optimized7 : dspsigops/NCO HDL Optimized  PhaseIncrementSource=Property  PhaseIncrement=-floor(4000*2^17/overSampleFreq)  PhaseOffsetSource=Property  PhaseOffset=0  DitherSource=Property  NumDitherBits=4  PhaseQuantization=on  NumQuantizerAccumulatorBits=17  LUTCompress=on  ResetAction=off  ValidInputPort=off  Waveform=Complex exponential  PhasePort=off  SimulateUsing=Code generation  AccumulatorWL=21  OutputDataType=Binary point scaling  OutputWL=18  OutputFL=11
      settings: SourceProductName=DSP System Toolbox  SourceProductBaseCode=DS
  NCO HDL Optimized8 : dspsigops/NCO HDL Optimized  PhaseIncrementSource=Property  PhaseIncrement=floor(5000*2^17/overSampleFreq)  PhaseOffsetSource=Property  PhaseOffset=0  DitherSource=Property  NumDitherBits=4  PhaseQuantization=on  NumQuantizerAccumulatorBits=17  LUTCompress=on  ResetAction=off  ValidInputPort=off  Waveform=Complex exponential  PhasePort=off  SimulateUsing=Code generation  AccumulatorWL=21  OutputDataType=Binary point scaling  OutputWL=18  OutputFL=11
      settings: SourceProductName=DSP System Toolbox  SourceProductBaseCode=DS
  NCO HDL Optimized9 : dspsigops/NCO HDL Optimized  PhaseIncrementSource=Property  PhaseIncrement=-floor(5000*2^17/overSampleFreq)  PhaseOffsetSource=Property  PhaseOffset=0  DitherSource=Property  NumDitherBits=4  PhaseQuantization=on  NumQuantizerAccumulatorBits=17  LUTCompress=on  ResetAction=off  ValidInputPort=off  Waveform=Complex exponential  PhasePort=off  SimulateUsing=Code generation  AccumulatorWL=21  OutputDataType=Binary point scaling  OutputWL=18  OutputFL=11
      settings: SourceProductName=DSP System Toolbox  SourceProductBaseCode=DS
  RxRaisedCosine : Subsystem
  RxRaisedCosine1 : Subsystem
  RxRaisedCosine10 : Subsystem
  RxRaisedCosine2 : Subsystem
  RxRaisedCosine3 : Subsystem
  RxRaisedCosine4 : Subsystem
  RxRaisedCosine5 : Subsystem
  RxRaisedCosine6 : Subsystem
  RxRaisedCosine7 : Subsystem
  RxRaisedCosine8 : Subsystem
  RxRaisedCosine9 : Subsystem
  Scope : Scope  NumInputPorts=11
  complex_magnitude_sq_cfg{,1..10} (11 alike) : helperLib/complex_magnitude_sq_cfg  mult=mult_pipeline  pipe=regular_pipeline
  pipelined_mult{1..10} (10 alike) : helperLib/pipelined_mult  d=wide_mult_pipeline
  Out1 : Outport
  wires:
  NCO HDL Optimized/1 -> pipelined_mult2/2
  NCO HDL Optimized1/1 -> pipelined_mult3/2
  pipelined_mult3/1 -> RxRaisedCosine2/1(In2)
  pipelined_mult2/1 -> RxRaisedCosine1/1(In2)
  NCO HDL Optimized6/1 -> pipelined_mult6/2
  NCO HDL Optimized4/1 -> pipelined_mult5/2
  NCO HDL Optimized2/1 -> pipelined_mult1/2
  pipelined_mult1/1 -> RxRaisedCosine3/1(In2)
  NCO HDL Optimized8/1 -> pipelined_mult7/2
  In1/1 -> Data Type Conversion/1
  NCO HDL Optimized3/1 -> pipelined_mult4/2
  NCO HDL Optimized5/1 -> pipelined_mult8/2
  NCO HDL Optimized7/1 -> pipelined_mult9/2
  NCO HDL Optimized9/1 -> pipelined_mult10/2
  pipelined_mult4/1 -> RxRaisedCosine4/1(In2)
  pipelined_mult8/1 -> RxRaisedCosine5/1(In2)
  pipelined_mult9/1 -> RxRaisedCosine6/1(In2)
  pipelined_mult10/1 -> RxRaisedCosine7/1(In2)
  pipelined_mult5/1 -> RxRaisedCosine8/1(In2)
  pipelined_mult6/1 -> RxRaisedCosine9/1(In2)
  pipelined_mult7/1 -> RxRaisedCosine10/1(In2)
  RxRaisedCosine10/1(Out2) -> complex_magnitude_sq_cfg/1
  RxRaisedCosine9/1(Out2) -> complex_magnitude_sq_cfg1/1
  RxRaisedCosine8/1(Out2) -> complex_magnitude_sq_cfg2/1
  RxRaisedCosine3/1(Out2) -> complex_magnitude_sq_cfg3/1
  RxRaisedCosine1/1(Out2) -> complex_magnitude_sq_cfg4/1
  RxRaisedCosine/1(Out2) -> complex_magnitude_sq_cfg5/1
  RxRaisedCosine2/1(Out2) -> complex_magnitude_sq_cfg6/1
  RxRaisedCosine4/1(Out2) -> complex_magnitude_sq_cfg7/1
  RxRaisedCosine5/1(Out2) -> complex_magnitude_sq_cfg8/1
  RxRaisedCosine6/1(Out2) -> complex_magnitude_sq_cfg9/1
  RxRaisedCosine7/1(Out2) -> complex_magnitude_sq_cfg10/1
  complex_magnitude_sq_cfg/1 -> Discrete FIR Filter/1
  complex_magnitude_sq_cfg1/1 -> Discrete FIR Filter1/1
  complex_magnitude_sq_cfg2/1 -> Discrete FIR Filter2/1
  complex_magnitude_sq_cfg3/1 -> Discrete FIR Filter3/1
  complex_magnitude_sq_cfg4/1 -> Discrete FIR Filter4/1
  complex_magnitude_sq_cfg5/1 -> Discrete FIR Filter5/1
  complex_magnitude_sq_cfg6/1 -> Discrete FIR Filter6/1
  complex_magnitude_sq_cfg7/1 -> Discrete FIR Filter7/1
  complex_magnitude_sq_cfg8/1 -> Discrete FIR Filter8/1
  complex_magnitude_sq_cfg9/1 -> Discrete FIR Filter9/1
  complex_magnitude_sq_cfg10/1 -> Discrete FIR Filter10/1
  Data Type Conversion/1 -> pipelined_mult7/1, pipelined_mult6/1, pipelined_mult5/1, pipelined_mult1/1, RxRaisedCosine/1(In2), pipelined_mult10/1, pipelined_mult9/1, pipelined_mult8/1, pipelined_mult4/1, pipelined_mult3/1, pipelined_mult2/1
  Discrete FIR Filter/1 -> Scope/1
  Discrete FIR Filter1/1 -> Scope/2
  Discrete FIR Filter2/1 -> Scope/3
  Discrete FIR Filter3/1 -> Scope/4
  Discrete FIR Filter4/1 -> Scope/5
  Discrete FIR Filter5/1 -> Scope/6
  Discrete FIR Filter6/1 -> Scope/7
  Discrete FIR Filter7/1 -> Scope/8
  Discrete FIR Filter8/1 -> Scope/9
  Discrete FIR Filter9/1 -> Scope/10
  Discrete FIR Filter10/1 -> Scope/11

== system rev0BB/receiver/slim_fast_rx2/coarseCFO_ff ==
  note: The frequency estemator is derived in Ch 8.2.2 (Pg 457-462) in
      | Digital Communication Recievers: Syncronization, Channel Estimation, and Signal Processing by Meyr et al.
  SignalIn : Inport
  Coarse_CFO_EST : Scope
  Complex to Real-Imag : ComplexToRealImag
  Constant : Constant  Value=0  OutDataTypeStr=int16
  Constant1 : Constant  Value=true  OutDataTypeStr=boolean
  Data Type Conversion : DataTypeConversion  OutDataTypeStr=double
  Data Type Conversion1 : DataTypeConversion  OutDataTypeStr=double
  Delay : Delay  DelayLength=1  InitialCondition=0
  Discrete FIR Filter : DiscreteFir  Coefficients=ones(1, 4096)  AccumDataTypeStr=Inherit: Same as product output
  Gain : Gain  Gain=overSampleFreq/(2*pi)
  NCO HDL Optimized : dspsigops/NCO HDL Optimized  PhaseIncrementSource=Input port  PhaseIncrement=100  PhaseOffsetSource=Property  PhaseOffset=0  DitherSource=Property  NumDitherBits=4  PhaseQuantization=on  NumQuantizerAccumulatorBits=12  LUTCompress=on  ResetAction=off  ValidInputPort=on  Waveform=Complex exponential  PhasePort=off  SimulateUsing=Code generation  AccumulatorWL=14  OutputDataType=Binary point scaling  OutputWL=14  OutputFL=11
      settings: SourceProductName=DSP System Toolbox  SourceProductBaseCode=DS
  Product : Product
  Trigonometric Function : Trigonometry  Operator=atan2
  complex_conj : helperLib/complex_conj
  pipeline_delay : Delay  DelayLength=regular_pipeline
  pipelined_mult1 : helperLib/pipelined_mult  d=wide_mult_pipeline
  SignalOut : Outport
  wires:
  NCO HDL Optimized/1 -> pipelined_mult1/2
  SignalIn/1 -> pipeline_delay/1, pipelined_mult1/1
  pipelined_mult1/1 -> SignalOut/1
  Constant1/1 -> NCO HDL Optimized/2
  Delay/1 -> complex_conj/1
  pipeline_delay/1 -> Data Type Conversion/1, Delay/1
  Constant/1 -> NCO HDL Optimized/1
  Trigonometric Function/1 -> Gain/1
  complex_conj/1 -> Data Type Conversion1/1
  Data Type Conversion1/1 -> Product/1
  Data Type Conversion/1 -> Product/2
  Product/1 -> Discrete FIR Filter/1
  Discrete FIR Filter/1 -> Complex to Real-Imag/1
  Complex to Real-Imag/2 -> Trigonometric Function/1
  Complex to Real-Imag/1 -> Trigonometric Function/2
  Gain/1 -> Coarse_CFO_EST/1

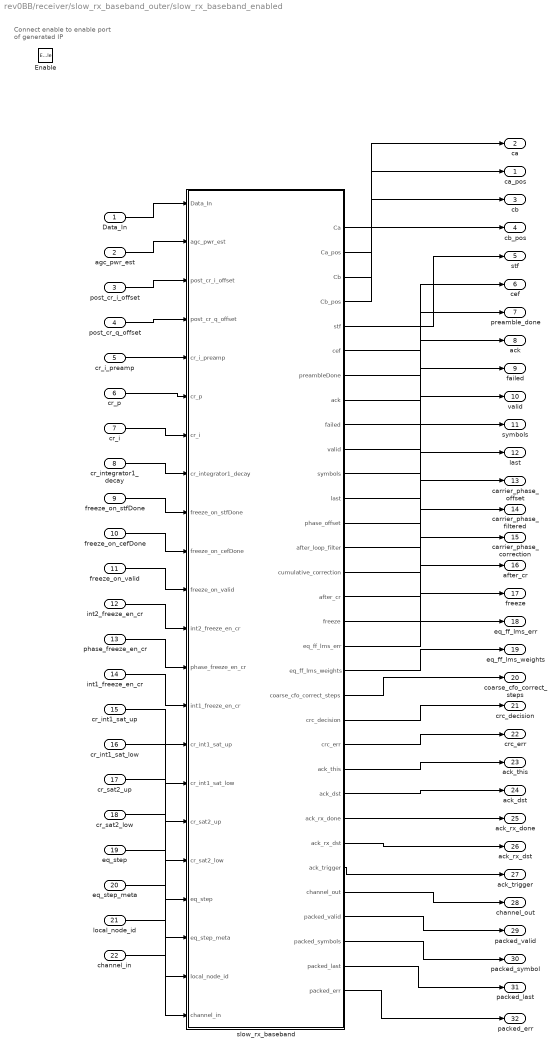
== system rev0BB/receiver/slow_rx_baseband_outer/slow_rx_baseband_enabled ==
  note: Connect enable to enable port of generated IP
  Data_In : Inport  SampleTime=slowPer
  agc_pwr_est : Inport  Port=2  SampleTime=slowPer
  post_cr_i_offset : Inport  Port=3
  post_cr_q_offset : Inport  Port=4
  cr_i_preamp : Inport  Port=5
  cr_p : Inport  Port=6
  cr_i : Inport  Port=7
  cr_integrator1_decay : Inport  Port=8
  freeze_on_stfDone : Inport  Port=9
  freeze_on_cefDone : Inport  Port=10
  freeze_on_valid : Inport  Port=11
  int2_freeze_en_cr : Inport  Port=12  OutDataTypeStr=boolean
  phase_freeze_en_cr : Inport  Port=13  OutDataTypeStr=boolean
  int1_freeze_en_cr : Inport  Port=14  OutDataTypeStr=boolean
  cr_int1_sat_up : Inport  Port=15
  cr_int1_sat_low : Inport  Port=16
  cr_sat2_up : Inport  Port=17
  cr_sat2_low : Inport  Port=18
  eq_step : Inport  Port=19
  eq_step_meta : Inport  Port=20
  local_node_id : Inport  Port=21
  channel_in : Inport  Port=22
  Enable : EnablePort
  slow_rx_baseband : Subsystem
  ca_pos : Outport  InitialOutput=0
  ca : Outport  Port=2  InitialOutput=0
  cb : Outport  Port=3  InitialOutput=0
  cb_pos : Outport  Port=4  InitialOutput=0
  stf : Outport  Port=5  InitialOutput=0
  cef : Outport  Port=6  InitialOutput=0
  preamble_done : Outport  Port=7  InitialOutput=0
  ack : Outport  Port=8  InitialOutput=0
  failed : Outport  Port=9  InitialOutput=0
  valid : Outport  Port=10  InitialOutput=0
  symbols : Outport  Port=11  InitialOutput=0
  last : Outport  Port=12  SampleTime=slowPer  InitialOutput=[0]
  carrier_phase_offset : Outport  Port=13  InitialOutput=0
  carrier_phase_filtered : Outport  Port=14  InitialOutput=0
  carrier_phase_correction : Outport  Port=15  InitialOutput=0
  after_cr : Outport  Port=16  InitialOutput=0
  freeze : Outport  Port=17  SampleTime=slowPer  InitialOutput=[0]
  eq_ff_lms_err : Outport  Port=18  SampleTime=slowPer  InitialOutput=0
  eq_ff_lms_weights : Outport  Port=19  SampleTime=slowPer  InitialOutput=0
  coarse_cfo_correct_steps : Outport  Port=20  SampleTime=slowPer  InitialOutput=0
  crc_decision : Outport  Port=21  SampleTime=slowPer  InitialOutput=0
  crc_err : Outport  Port=22  SampleTime=slowPer  InitialOutput=0
  ack_this : Outport  Port=23  SampleTime=slowPer  InitialOutput=0
  ack_dst : Outport  Port=24  SampleTime=slowPer  InitialOutput=0
  ack_rx_done : Outport  Port=25  SampleTime=slowPer  InitialOutput=0
  ack_rx_dst : Outport  Port=26  SampleTime=slowPer  InitialOutput=0
  ack_trigger : Outport  Port=27  SampleTime=slowPer  InitialOutput=0
  channel_out : Outport  Port=28  SampleTime=slowPer  InitialOutput=0
  packed_valid : Outport  Port=29  SampleTime=slowPer  InitialOutput=0
  packed_symbol : Outport  Port=30  SampleTime=slowPer  InitialOutput=0
  packed_last : Outport  Port=31  SampleTime=slowPer  InitialOutput=0
  packed_err : Outport  Port=32  SampleTime=slowPer  InitialOutput=0
  wires:
  slow_rx_baseband/1(Ca) -> ca/1
  slow_rx_baseband/2(Ca_pos) -> ca_pos/1
  slow_rx_baseband/3(Cb) -> cb/1
  slow_rx_baseband/4(Cb_pos) -> cb_pos/1
  slow_rx_baseband/5(stf) -> stf/1
  slow_rx_baseband/6(cef) -> cef/1
  slow_rx_baseband/7(preambleDone) -> preamble_done/1
  slow_rx_baseband/9(failed) -> failed/1
  slow_rx_baseband/10(valid) -> valid/1
  slow_rx_baseband/11(symbols) -> symbols/1
  slow_rx_baseband/13(phase_offset) -> carrier_phase_offset/1
  slow_rx_baseband/14(after_loop_filter) -> carrier_phase_filtered/1
  slow_rx_baseband/15(cumulative_correction) -> carrier_phase_correction/1
  Data_In/1 -> slow_rx_baseband/1(Data_In)
  slow_rx_baseband/16(after_cr) -> after_cr/1
  post_cr_i_offset/1 -> slow_rx_baseband/3(post_cr_i_offset)
  post_cr_q_offset/1 -> slow_rx_baseband/4(post_cr_q_offset)
  cr_i_preamp/1 -> slow_rx_baseband/5(cr_i_preamp)
  cr_p/1 -> slow_rx_baseband/6(cr_p)
  cr_i/1 -> slow_rx_baseband/7(cr_i)
  cr_integrator1_decay/1 -> slow_rx_baseband/8(cr_integrator1_decay)
  freeze_on_stfDone/1 -> slow_rx_baseband/9(freeze_on_stfDone)
  freeze_on_cefDone/1 -> slow_rx_baseband/10(freeze_on_cefDone)
  freeze_on_valid/1 -> slow_rx_baseband/11(freeze_on_valid)
  slow_rx_baseband/17(freeze) -> freeze/1
  int2_freeze_en_cr/1 -> slow_rx_baseband/12(int2_freeze_en_cr)
  cr_int1_sat_up/1 -> slow_rx_baseband/15(cr_int1_sat_up)
  cr_int1_sat_low/1 -> slow_rx_baseband/16(cr_int1_sat_low)
  cr_sat2_up/1 -> slow_rx_baseband/17(cr_sat2_up)
  cr_sat2_low/1 -> slow_rx_baseband/18(cr_sat2_low)
  phase_freeze_en_cr/1 -> slow_rx_baseband/13(phase_freeze_en_cr)
  int1_freeze_en_cr/1 -> slow_rx_baseband/14(int1_freeze_en_cr)
  slow_rx_baseband/12(last) -> last/1
  slow_rx_baseband/18(eq_ff_lms_err) -> eq_ff_lms_err/1
  agc_pwr_est/1 -> slow_rx_baseband/2(agc_pwr_est)
  eq_step/1 -> slow_rx_baseband/19(eq_step)
  eq_step_meta/1 -> slow_rx_baseband/20(eq_step_meta)
  slow_rx_baseband/19(eq_ff_lms_weights) -> eq_ff_lms_weights/1
  slow_rx_baseband/20(coarse_cfo_correct_steps) -> coarse_cfo_correct_steps/1
  slow_rx_baseband/21(crc_decision) -> crc_decision/1
  slow_rx_baseband/22(crc_err) -> crc_err/1
  local_node_id/1 -> slow_rx_baseband/21(local_node_id)
  slow_rx_baseband/23(ack_this) -> ack_this/1
  slow_rx_baseband/24(ack_dst) -> ack_dst/1
  slow_rx_baseband/8(ack) -> ack/1
  slow_rx_baseband/25(ack_rx_done) -> ack_rx_done/1
  slow_rx_baseband/26(ack_rx_dst) -> ack_rx_dst/1
  slow_rx_baseband/27(ack_trigger) -> ack_trigger/1
  channel_in/1 -> slow_rx_baseband/22(channel_in)
  slow_rx_baseband/28(channel_out) -> channel_out/1
  slow_rx_baseband/29(packed_valid) -> packed_valid/1
  slow_rx_baseband/30(packed_symbols) -> packed_symbol/1
  slow_rx_baseband/31(packed_last) -> packed_last/1
  slow_rx_baseband/32(packed_err) -> packed_err/1

== system rev0BB/transmitter/transmitter_internal/Tx_LPF ==
  In1 : Inport
  TxLPF_Filter : DiscreteFir  FilterStructure=Direct form transposed  Coefficients=txLPF_coef  OutDataTypeStr=Inherit: Same as input
  Out1 : Outport
  wires:
  In1/1 -> TxLPF_Filter/1
  TxLPF_Filter/1 -> Out1/1

== system rev0BB/transmitter/transmitter_internal/raised_cosine ==
  note: (a+bj)(c+dj) = ac+adj+bcj-bd
      | If d = 0 | = ac + bcj
  note: Raised Cosine Filter Can be Split because it is Real (use 2 multiplies instead of 4 per tap)
  note: Note: the tool should optomize a single FIR filter to this config due to 0 propogation. However, will make explicit for now
  In1 : Inport
  Discrete FIR Filter : DiscreteFir  FilterStructure=Direct form transposed  Coefficients=rcTxFilt
  Raised Cosine Transmit Filter : commfilt2/Raised Cosine Transmit Filter  Commented=on  filtType=Square root  R=.1  filtSpan=30  N=4  filterGain=1  RateOptions=Allow multirate processing  framing=Mute  checkCoeff=on  variableName=rcTxFilt  checkGain=Normalized  sampMode=Mute  saveAsFlag=0  currentFiltSpan=30  D=(30)/2  launchFVT=on  roundingMode=Floor  overflowMode=off  coeffDataTypeStr=Inherit: Same word length as input  coeffMin=[]  coeffMax=[]  coeffLastDataTypeStr=Inherit: Same word length as input  outputDataTypeStr=Inherit: Same as accumulator  outputMin=[]  outputMax=[]  outputLastDataTypeStr=Inherit: Same as accumulator
  Raised Cosine Transmit Filter_full : commfilt2/Raised Cosine Transmit Filter  Commented=on  filtType=Normal  R=0.08  filtSpan=40  N=4  filterGain=1  RateOptions=Allow multirate processing  framing=Mute  checkCoeff=on  variableName=rcTxFilt_full  checkGain=Normalized  sampMode=Mute  saveAsFlag=0  currentFiltSpan=40  D=(40)/2  launchFVT=on  roundingMode=Floor  overflowMode=off  coeffDataTypeStr=Inherit: Same word length as input  coeffMin=[]  coeffMax=[]  coeffLastDataTypeStr=Inherit: Same word length as input  outputDataTypeStr=Inherit: Same as accumulator  outputMin=[]  outputMax=[]  outputLastDataTypeStr=Inherit: Same as accumulator
  mult_delay : Delay  DelayLength=mult_pipeline
  mult_delay1 : Delay  DelayLength=mult_pipeline
  Out1 : Outport
  wires:
  In1/1 -> mult_delay/1
  mult_delay/1 -> Discrete FIR Filter/1
  mult_delay1/1 -> Out1/1
  Discrete FIR Filter/1 -> mult_delay1/1

== system rev0BB/transmitter/transmitter_internal/zero_fill_counter ==
  Compare To Constant : simulink/Logic and Bit Operations/Compare To Constant  relop=>=  const=3  OutDataTypeStr=boolean
  Constant2 : Constant  OutDataTypeStr=uint8  SampleTime=-1
  Constant3 : Constant  Value=0  OutDataTypeStr=uint8  SampleTime=-1
  Delay : Delay  DelayLength=1  InitialCondition=0
  Sum : Sum  Inputs=|++  OutDataTypeStr=Inherit: Same as first input
  Switch1 : Switch  Criteria=u2 > Threshold
  Out1 : Outport
  wires:
  Switch1/1 -> Delay/1
  Compare To Constant/1 -> Switch1/2
  Constant3/1 -> Switch1/1
  Delay/1 -> Out1/1, Sum/2, Compare To Constant/1
  Constant2/1 -> Sum/1
  Sum/1 -> Switch1/3
